simulink model "Demand"  (R2024b)
settings: Solver=VariableStepAuto  StartTime=0.0  StopTime=365*24  RelTol=1e-3
libraries: Demand_lib x1
settings Model: Creator=20223126  LastModifiedBy=20223126
settings DataIOCC: SaveFormat=Array

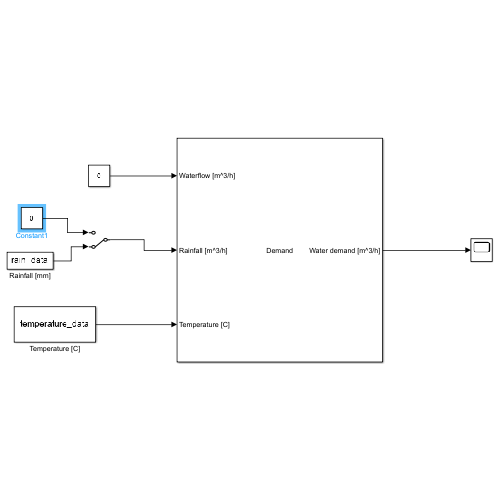
[thumbnail: Simulink's stored preview of the top-level diagram]
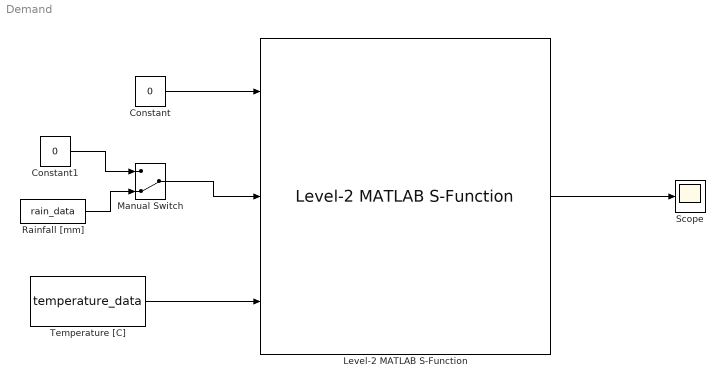
== system Demand ==
  Constant : Constant  Value=0
  Constant1 : Constant  Value=0
  Level-2 MATLAB S-Function : Demand_lib/Level-2 MATLAB S-Function  Type_demand=Agriculture  Constant_demand=3e5  Crop_type=Potato  Area=1e5  Type_soil=Clay soil  Type_control=Normal control  Predictive_steps=10
  Manual Switch : ManualSwitch  CurrentSetting=0
  Rainfall [mm] : FromWorkspace  VariableName=rain_data  OutDataTypeStr=double  SampleTime=1
  Scope : Scope
  Temperature [C] : FromWorkspace  VariableName=temperature_data  OutDataTypeStr=double  SampleTime=1
  wires:
  Level-2 MATLAB S-Function/1 -> Scope/1
  Constant/1 -> Level-2 MATLAB S-Function/1
  Rainfall [mm]/1 -> Manual Switch/2
  Constant1/1 -> Manual Switch/1
  Temperature [C]/1 -> Level-2 MATLAB S-Function/3
  Manual Switch/1 -> Level-2 MATLAB S-Function/2
